simulink model "PI_controller"  (R2023a)
settings: Solver=VariableStepAuto  StartTime=0.0  StopTime=10.0  RelTol=1e-3
model workspace (MAT data in the model file):
  Ki = 2
  Kp = 0.3
  Ts = 0.01
settings Model: Creator=Administrator  LastModifiedBy=Administrator

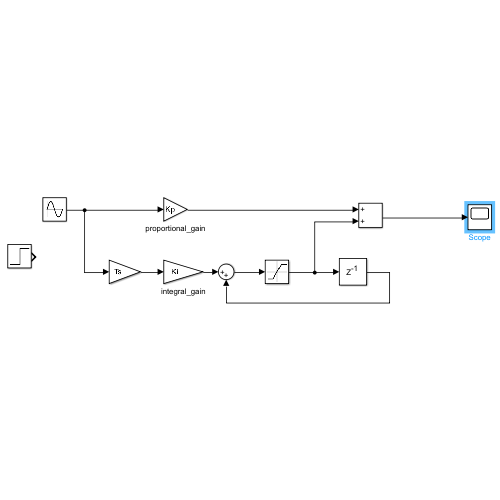
[thumbnail: Simulink's stored preview of the top-level diagram]
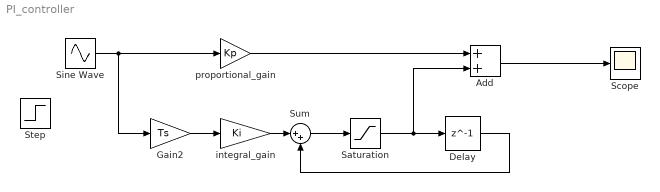
== system PI_controller ==
  Add : Sum
  Delay : Delay  DelayLength=1  InitialCondition=0  SampleTime=0.01
  Gain2 : Gain  Gain=Ts
  Saturation : Saturate  UpperLimit=1  LowerLimit=-1
  Scope : Scope
  Sine Wave : Sin  Amplitude=0.5  Frequency=10  SampleTime=0
  Step : Step  SampleTime=0
  Sum : Sum  Inputs=|++
  integral_gain : Gain  Gain=Ki
  proportional_gain : Gain  Gain=Kp
  wires:
  Gain2/1 -> integral_gain/1
  integral_gain/1 -> Sum/1
  proportional_gain/1 -> Add/1
  Add/1 -> Scope/1
  Saturation/1 -> Delay/1, Add/2
  Sum/1 -> Saturation/1
  Delay/1 -> Sum/2
  Sine Wave/1 -> Gain2/1, proportional_gain/1
